simulink model "simulink_lineare"  (R2025b)
settings: Solver=ode45  StartTime=0.0  StopTime=0.5  MaxStep=1e-4  RelTol=1e-3
values from neighbouring files (symbols this model uses):
  A = [ -k1/(2*sqrt(x1e)),      0 ... (first row only)    [main.m]
  alpha = alpha_tau / tau    [main.m]
  B = [ k4; 0 ]    [main.m]
  C = [ 0, 1 ]    [main.m]
  D = 0    [main.m]
  tau = (M_star - cos(phi_rad)) / (wc_des * sin(phi_rad))    [main.m]
undefined symbols (not defined in the file or in its folder): Kr
settings Model: Creator=porpo  LastModifiedBy=porpo

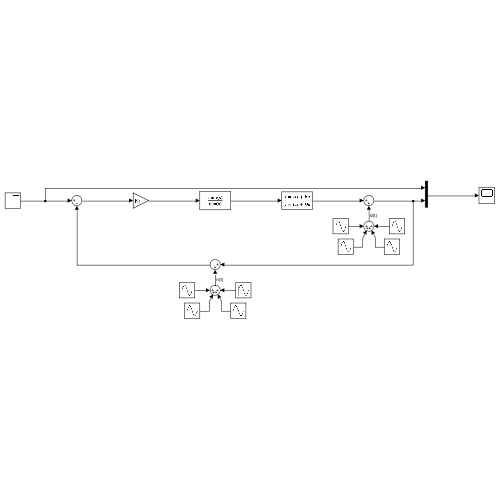
[thumbnail: Simulink's stored preview of the top-level diagram]
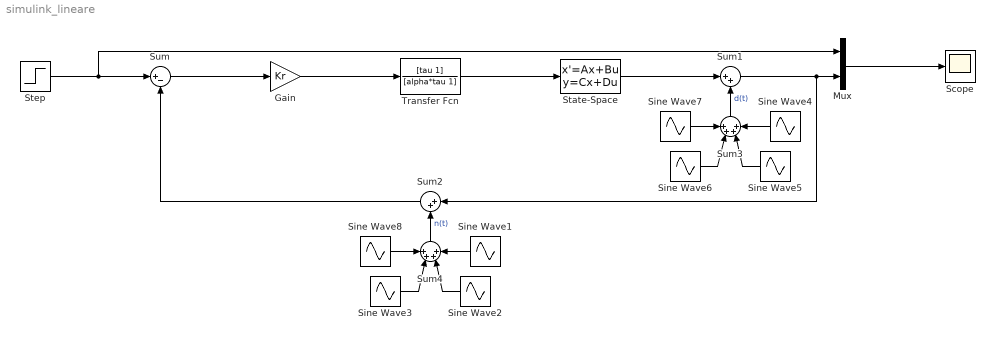
== system simulink_lineare ==
  Gain : Gain  Gain=Kr
  Mux : Mux  Inputs=2
  Scope : Scope
      settings: ActiveDisplayYMinimum=3.1114544562900983  ActiveDisplayYMaximum=3.1472114586953417
  Sine Wave1 : Sin  Amplitude=2.5  Frequency=1e5*1  SampleTime=0
  Sine Wave2 : Sin  Amplitude=2.5  Frequency=1e5*2  SampleTime=0
  Sine Wave3 : Sin  Amplitude=2.5  Frequency=1e5*3  SampleTime=0
  Sine Wave4 : Sin  Frequency=0.4  SampleTime=0
  Sine Wave5 : Sin  Frequency=0.3  SampleTime=0
  Sine Wave6 : Sin  Frequency=0.2  SampleTime=0
  Sine Wave7 : Sin  Frequency=0.1  SampleTime=0
  Sine Wave8 : Sin  Amplitude=2.5  Frequency=1e5*4  SampleTime=0
  State-Space : StateSpace  A=A  B=B  C=C  D=D  InitialCondition=0
  Step : Step  Time=0  After=3  SampleTime=0
  Sum : Sum  Inputs=|+-
  Sum1 : Sum  Inputs=|++
  Sum2 : Sum  Inputs=|++
  Sum3 : Sum  Inputs=++++
  Sum4 : Sum  Inputs=++++
  Transfer Fcn : TransferFcn  Numerator=[tau 1]  Denominator=[alpha*tau 1]
  wires:
  Step/1 -> Mux/1, Sum/1
  Sum/1 -> Gain/1
  Gain/1 -> Transfer Fcn/1
  Transfer Fcn/1 -> State-Space/1
  State-Space/1 -> Sum1/1
  Sum1/1 -> Mux/2, Sum2/1
  Sum2/1 -> Sum/2
  Mux/1 -> Scope/1
  Sine Wave7/1 -> Sum3/1
  Sine Wave5/1 -> Sum3/3
  Sine Wave4/1 -> Sum3/4
  Sine Wave6/1 -> Sum3/2
  Sum3/1 -> Sum1/2  "d(t)"
  Sum4/1 -> Sum2/2  "n(t)"
  Sine Wave1/1 -> Sum4/4
  Sine Wave2/1 -> Sum4/3
  Sine Wave3/1 -> Sum4/2
  Sine Wave8/1 -> Sum4/1
